simulink model "LabSimulation"  (R2022a)
settings: Solver=VariableStepAuto  StartTime=0.0  StopTime=6  RelTol=1e-3
libraries: slpidlib x1, simulink x1
settings Model: Creator=sarah  LastModifiedBy=sarah
settings DebuggingCC: UnconnectedInputMsg=warning  UnconnectedOutputMsg=warning  UnconnectedLineMsg=warning
settings RTWCC: DLArmComputeVersion=19.05

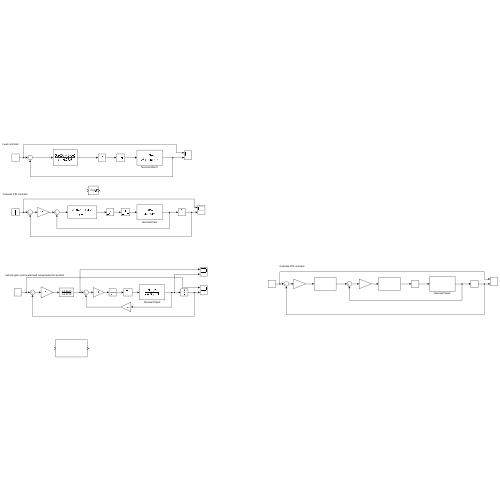
[thumbnail: Simulink's stored preview of the top-level diagram]
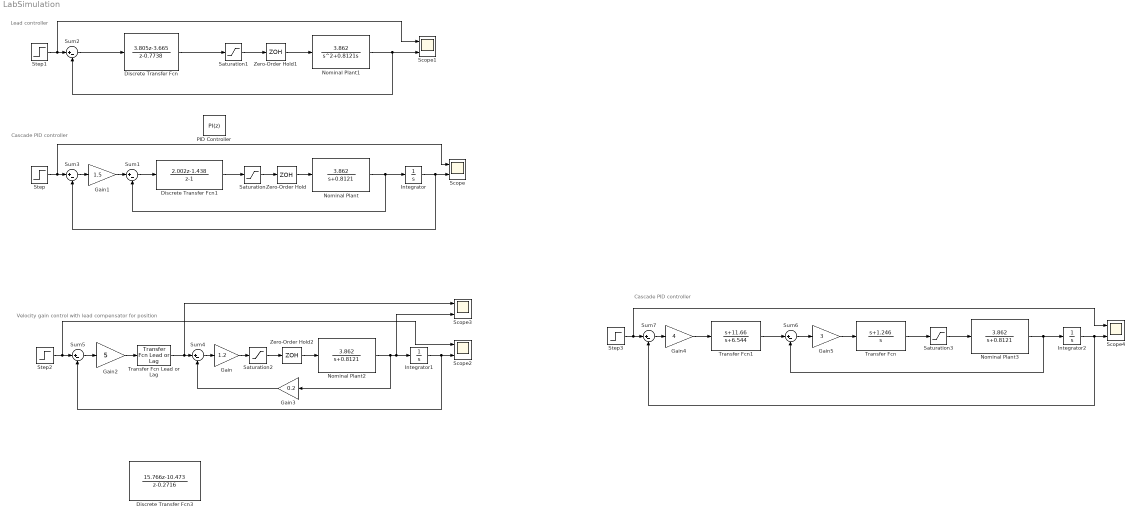
== system LabSimulation ==
  note: Cascade PID controller
  note: Lead controller
  note: Velocity gain control with lead compensator for position
  note: Cascade PID controller
  Discrete Transfer Fcn : DiscreteTransferFcn  Numerator=[3.805 -3.665]  Denominator=[1 -0.7738]
  Discrete Transfer Fcn1 : DiscreteTransferFcn  Numerator=[2.002 -1.438]  Denominator=[1 -1]  SampleTime=0.05
  Discrete Transfer Fcn3 : DiscreteTransferFcn  Numerator=[15.766 -10.473]  Denominator=[1 -0.2716]
  Gain : Gain  Gain=1.2
  Gain1 : Gain  Gain=1.5
  Gain2 : Gain  Gain=5
  Gain3 : Gain  Gain=0.2
  Gain4 : Gain  Gain=4
  Gain5 : Gain  Gain=3
  Integrator : Integrator
  Integrator1 : Integrator
  Integrator2 : Integrator
  Nominal Plant : TransferFcn  Numerator=[3.862]  Denominator=[1 0.8121]
  Nominal Plant1 : TransferFcn  Numerator=[3.862]  Denominator=[1 0.8121 0]
  Nominal Plant2 : TransferFcn  Numerator=[3.862]  Denominator=[1 0.8121]
  Nominal Plant3 : TransferFcn  Numerator=[3.862]  Denominator=[1 0.8121]
  PID Controller : slpidlib/PID Controller  Controller=PI  Form=Parallel  TimeDomain=Discrete-time  UseExternalTs=off  SampleTime=0.05  IntegratorMethod=Forward Euler  FilterMethod=Forward Euler  ControllerParametersSource=internal  P=1.72  I=5.65  UseKiTs=off  D=0  N=100  UseFilter=on  TunerSelectOption=Transfer Function Based (PID Tuner App)  InitialConditionSource=internal  InitialConditionForIntegrator=0  InitialConditionForFilter=0  DifferentiatorICPrevScaledInput=0  ExternalReset=none  TrackingMode=off  Kt=1  LimitOutput=on  SatLimitsSource=internal  UpperSaturationLimit=10  LowerSaturationLimit=-10  LinearizeAsGain=on  AntiWindupMode=none  Kb=1  POutMin=[]  POutMax=[]  IOutMin=[]  IOutMax=[]  DOutMin=[]  DOutMax=[]  NOutMin=[]  NOutMax=[]  SumOutMin=[]  SumOutMax=[]  SaturationOutMin=[]  SaturationOutMax=[]  PParamMin=[]  PParamMax=[]  IParamMin=[]  IParamMax=[]  DParamMin=[]  DParamMax=[]  NParamMin=[]  NParamMax=[]  KbParamMin=[]  KbParamMax=[]  KtParamMin=[]  KtParamMax=[]  KbOutMin=[]  KbOutMax=[]  KtOutMin=[]  KtOutMax=[]  IntegratorOutMin=[]  IntegratorOutMax=[]  FilterOutMin=[]  FilterOutMax=[]  SumI1OutMin=[]  SumI1OutMax=[]  SumI2OutMin=[]  SumI2OutMax=[]  SumI3OutMin=[]  SumI3OutMax=[]  SumI4OutMin=[]  SumI4OutMax=[]  SumDOutMin=[]  SumDOutMax=[]  DifferentiatorOutMin=[]  DifferentiatorOutMax=[]  FilterDiffOutCoefMin=[]  FilterDiffOutCoefMax=[]  ReciprocalOutMin=[]  ReciprocalOutMax=[]  SumDenOutMin=[]  SumDenOutMax=[]  SumNumOutMin=[]  SumNumOutMax=[]  DivideOutMin=[]  DivideOutMax=[]  UdiffTsProdOutMin=[]  UdiffTsProdOutMax=[]  NTsProdOutMin=[]  NTsProdOutMax=[]  UintegralTsProdOutMin=[]  UintegralTsProdOutMax=[]  UngainTsProdOutMin=[]  UngainTsProdOutMax=[]  IntegratorContinuousStateAttributes=''  IntegratorStateMustResolveToSignalObject=off  IntegratorRTWStateStorageClass=Auto  FilterContinuousStateAttributes=''  FilterStateMustResolveToSignalObject=off  FilterRTWStateStorageClass=Auto  ParallelPVariant=InternalParameters  IdealPVariant=Disabled  IVariant=InternalParameters  DVariant=Disabled  IntegratorVariant=Discrete  SatVariant=Enabled  AWVariant=Passthrough  PCopyVariant=Disabled  TRVariant=Disabled  FdbkBlocksVariant=Forward  IdealPFdbkVariant=Disabled  SatFdbkVariant=Disabled  DerivativeFilterVariant=Disabled  NVariant=Disabled  NCopyVariant=Disabled_SignalSpec  FilterICVariant=Disabled  IntegratorICVariant=InternalICs  ExternalResetVariant=Disabled  TRSumVariant=Passthrough  SumFdbkVariant=Disabled  SumVariant=Sum_PI  TsampFilterVariant=InternalTs  TsampNgainVariant=Passthrough  TsampIntegralVariant=Passthrough  ExternalSaturationOutDataTypeStr=Inherit: Same as second input  aMode=0
  Saturation{,1..3} (4 alike) : Saturate  UpperLimit=+10  LowerLimit=-10
  Scope{,1..4} (5 alike) : Scope  NumInputPorts=2
  Step{,1..3} (4 alike) : Step  After=5  SampleTime=0
  Sum{1..7} (7 alike) : Sum  Inputs=|+-
  Transfer Fcn : TransferFcn  Numerator=[1 1.246]  Denominator=[1 0]
  Transfer Fcn Lead or Lag : simulink/Discrete/Transfer Fcn Lead or Lag  PoleZ=0.2716  ZeroZ=0.6643  ICPrevOutput=0.0  ICPrevInput=0.0  DoSatur=off
      settings: SourceProductBaseCode=SL
  Transfer Fcn1 : TransferFcn  Numerator=[1 11.66]  Denominator=[1 6.544]
  Zero-Order Hold : ZeroOrderHold  SampleTime=0.05
  Zero-Order Hold1 : ZeroOrderHold  SampleTime=0.02
  Zero-Order Hold2 : ZeroOrderHold  SampleTime=0.1
  wires:
  Nominal Plant1/1 -> Scope1/2, Sum2/2
  Sum2/1 -> Discrete Transfer Fcn/1
  Saturation1/1 -> Zero-Order Hold1/1
  Step1/1 -> Scope1/1, Sum2/1
  Zero-Order Hold1/1 -> Nominal Plant1/1
  Discrete Transfer Fcn/1 -> Saturation1/1
  Sum3/1 -> Gain1/1
  Gain1/1 -> Sum1/1
  Nominal Plant/1 -> Sum1/2, Integrator/1
  Zero-Order Hold/1 -> Nominal Plant/1
  Step/1 -> Sum3/1, Scope/1
  Saturation/1 -> Zero-Order Hold/1
  Integrator/1 -> Sum3/2, Scope/2
  Sum1/1 -> Discrete Transfer Fcn1/1
  Discrete Transfer Fcn1/1 -> Saturation/1
  Saturation2/1 -> Zero-Order Hold2/1
  Step2/1 -> Sum5/1, Scope2/1
  Zero-Order Hold2/1 -> Nominal Plant2/1
  Nominal Plant2/1 -> Gain3/1, Scope3/2, Integrator1/1
  Integrator1/1 -> Sum5/2, Scope2/2
  Gain/1 -> Saturation2/1
  Sum4/1 -> Gain/1
  Gain3/1 -> Sum4/2
  Sum5/1 -> Gain2/1
  Gain2/1 -> Transfer Fcn Lead or Lag/1
  Transfer Fcn Lead or Lag/1 -> Scope3/1, Sum4/1
  Transfer Fcn/1 -> Saturation3/1
  Sum6/1 -> Gain5/1
  Step3/1 -> Sum7/1, Scope4/1
  Saturation3/1 -> Nominal Plant3/1
  Gain4/1 -> Transfer Fcn1/1
  Sum7/1 -> Gain4/1
  Nominal Plant3/1 -> Sum6/2, Integrator2/1
  Integrator2/1 -> Sum7/2, Scope4/2
  Gain5/1 -> Transfer Fcn/1
  Transfer Fcn1/1 -> Sum6/1
